simulink model "lorenz_sim"  (R2021a)
settings: Solver=VariableStepAuto  StartTime=0.0  StopTime=10.0  RelTol=1e-3
values from neighbouring files (symbols this model uses):
  K = lqr(A,B,Q,R)    [design.m]    (also in lorenz_system_lqr.m)
undefined symbols (not defined in the file or in its folder): beta, rho, sigma, x0
settings Model: Creator=toure  LastModifiedBy=toure

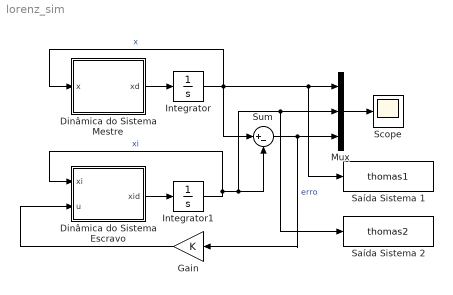
== system lorenz_sim ==
  Dinâmica do Sistema Escravo : MATLAB Function  TreatAsAtomicUnit=on
  Dinâmica do Sistema Mestre : MATLAB Function  TreatAsAtomicUnit=on
  Gain : Gain  Gain=K
  Integrator : Integrator  InitialCondition=x0
  Integrator1 : Integrator  InitialCondition=13*x0
  Mux : Mux  Inputs=3
  Saída Sistema 1 : ToWorkspace  VariableName=thomas1  SaveFormat=Timeseries  SampleTime=-1
      settings: Save2DSignal=2-D array (concatenate along first dimension)
  Saída Sistema 2 : ToWorkspace  VariableName=thomas2  SaveFormat=Timeseries  SampleTime=-1
      settings: Save2DSignal=2-D array (concatenate along first dimension)
  Scope : Scope
  Sum : Sum  Inputs=|+-
  wires:
  Integrator/1 -> Dinâmica do Sistema Mestre/1(x), Sum/1, Saída Sistema 1/1, Mux/1  "x"
  Sum/1 -> Gain/1, Mux/3  "erro"
  Dinâmica do Sistema Escravo/1(xid) -> Integrator1/1
  Integrator1/1 -> Saída Sistema 2/1, Mux/2, Sum/2, Dinâmica do Sistema Escravo/1(xi)  "xi"
  Mux/1 -> Scope/1
  Dinâmica do Sistema Mestre/1(xd) -> Integrator/1
  Gain/1 -> Dinâmica do Sistema Escravo/2(u)

== matlab function lorenz_sim/Dinâmica do Sistema Escravo ==
  data: xi input; u input; xid output; sigma parameter; rho parameter; beta parameter
function xid = fcn(xi,u,sigma,rho, beta)

xid = [sigma*(xi(2) - xi(1)) + u(1)
       (rho - xi(3))*xi(1) - xi(2) + u(2)
       xi(1)*xi(2) - beta*xi(3) + u(3)];
end

== matlab function lorenz_sim/Dinâmica do Sistema Mestre ==
  data: x input; xd output; sigma parameter; rho parameter; beta parameter
function xd = fcn(x,sigma,rho, beta)

xd = [sigma*(x(2)-x(1))
      (rho - x(3))*x(1) - x(2)
      x(1)*x(2) - beta*x(3)];
end
